simulink model "system2_net"  (R2019b)
settings: Solver=VariableStepAuto  StartTime=0.0  StopTime=10.0  RelTol=1e-3
settings Model: Creator=davis  LastModifiedBy=davis

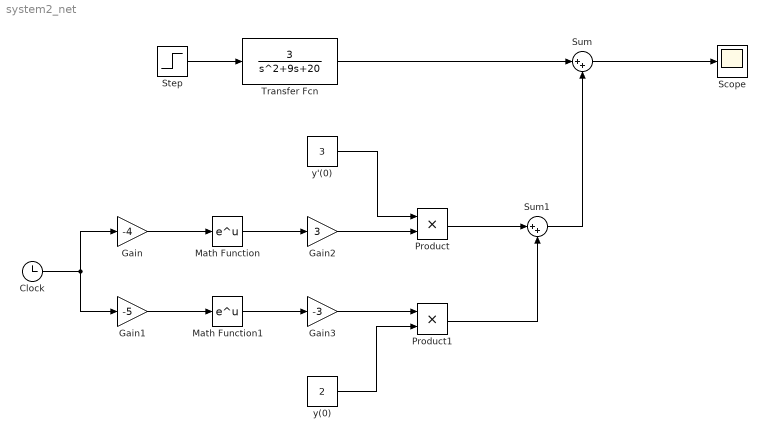
== system system2_net ==
  " y'(0)" : Constant  Value=3
  " y(0)" : Constant  Value=2
  Clock : Clock
  Gain : Gain  Gain=-4
  Gain1 : Gain  Gain=-5
  Gain2 : Gain  Gain=3
  Gain3 : Gain  Gain=-3
  Math Function : Math  SignedPower=off  SaturateOnIntegerOverflow=on
  Math Function1 : Math  SignedPower=off  SaturateOnIntegerOverflow=on
  Product : Product
  Product1 : Product
  Scope : Scope
  Step : Step  SampleTime=0
  Sum : Sum  Inputs=|++
  Sum1 : Sum  Inputs=|++
  Transfer Fcn : TransferFcn  Numerator=[3]  Denominator=[1 9 20]
  wires:
  Clock/1 -> Gain1/1, Gain/1
  Gain/1 -> Math Function/1
  Gain1/1 -> Math Function1/1
  Math Function1/1 -> Gain3/1
  Math Function/1 -> Gain2/1
  " y(0)"/1 -> Product1/2
  Gain3/1 -> Product1/1
  " y'(0)"/1 -> Product/1
  Gain2/1 -> Product/2
  Product/1 -> Sum1/1
  Product1/1 -> Sum1/2
  Transfer Fcn/1 -> Sum/1
  Sum1/1 -> Sum/2
  Step/1 -> Transfer Fcn/1
  Sum/1 -> Scope/1
